simulink model "carmodel_tesla"  (R2018a)
settings: Solver=VariableStepAuto  StartTime=0.0  StopTime=10.0  RelTol=1e-3
settings Model: Creator=abc  LastModifiedBy=abc

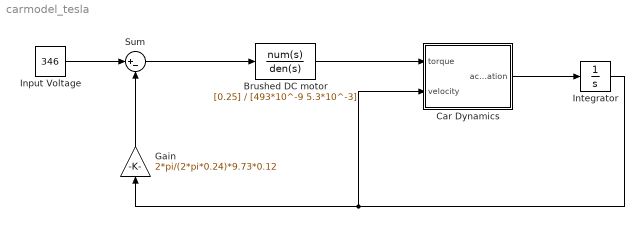
== system carmodel_tesla ==
  Brushed DC motor : TransferFcn  Numerator=[0.25]  Denominator=[493*10^-9 5.3*10^-3]
  Car Dynamics : MATLAB Function  TreatAsAtomicUnit=on
  Gain : Gain  Gain=2*pi/(2*pi*0.24)*9.73*0.12
  Input Voltage : Constant  Value=346
  Integrator : Integrator
  Sum : Sum  Inputs=|+-
  wires:
  Input Voltage/1 -> Sum/1
  Gain/1 -> Sum/2
  Sum/1 -> Brushed DC motor/1
  Brushed DC motor/1 -> Car Dynamics/1(torque)
  Car Dynamics/1(acceleration) -> Integrator/1
  Integrator/1 -> Gain/1, Car Dynamics/2(velocity)

== matlab function carmodel_tesla/Car Dynamics ==
  data: torque input; acceleration output; velocity input
function acceleration = fn(torque,velocity)
acceleration = (40.5*Torque*0.7-413-0.3381*velocity^2)/2108;
